simulink model "untitled1"  (R2025b)
settings: Solver=VariableStepAuto  StartTime=0.0  StopTime=10.0  RelTol=1e-3
settings Model: Creator=Hp  LastModifiedBy=Hp

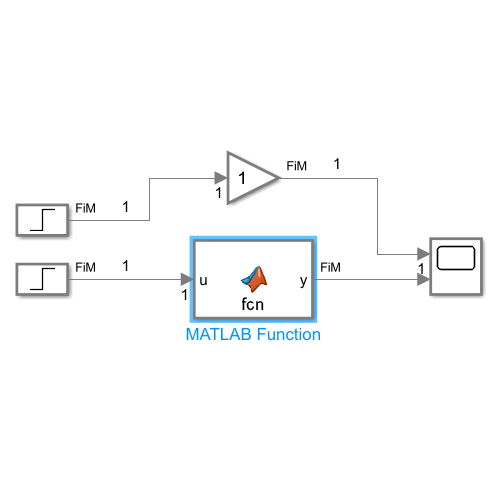
[thumbnail: Simulink's stored preview of the top-level diagram]
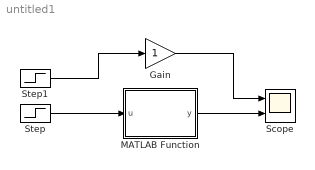
== system untitled1 ==
  Gain : Gain
  MATLAB Function : MATLAB Function  TreatAsAtomicUnit=on
  Scope : Scope  NumInputPorts=2
      settings: ActiveDisplayYMinimum=-11.46755633529294  ActiveDisplayYMaximum=4.9119553878685451
  Step : Step  SampleTime=0
  Step1 : Step  SampleTime=0
  wires:
  Step/1 -> MATLAB Function/1(u)
  MATLAB Function/1(y) -> Scope/2
  Step1/1 -> Gain/1
  Gain/1 -> Scope/1

== matlab function untitled1/MATLAB Function ==
  data: u input; y output
function y = fcn(u)

persistent p

if isempty(p)
    data = load('mlmodel3.mat');
    p = data.p;
end

y = polyval(p, u);

end
